simulink model "RLC3rdOrder"  (R2023b)
settings: Solver=VariableStepAuto  StartTime=0.0  StopTime=10.0  RelTol=1e-3
values from neighbouring files (symbols this model uses):
  C = 15    [SimScript.m]
  E = 575    [SimScript.m]
  Kd = 33    [SimScript.m]
  Ki = 10    [SimScript.m]
  Kp = 18    [SimScript.m]
  L = 10    [SimScript.m]
  Q = 10000    [SimScript.m]
  Q0 = 0    [SimScript.m]
  R = 100    [SimScript.m]
settings Model: Creator=Owner  LastModifiedBy=Owner

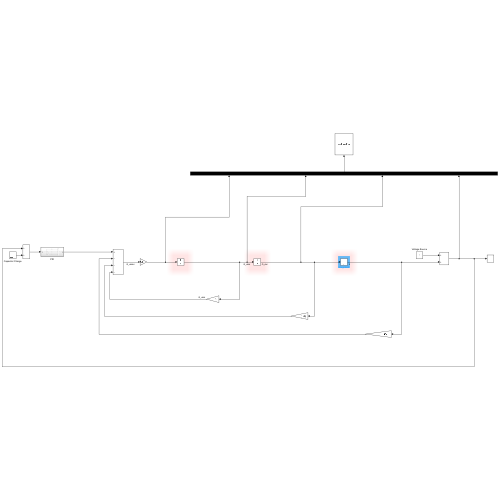
[thumbnail: Simulink's stored preview of the top-level diagram]
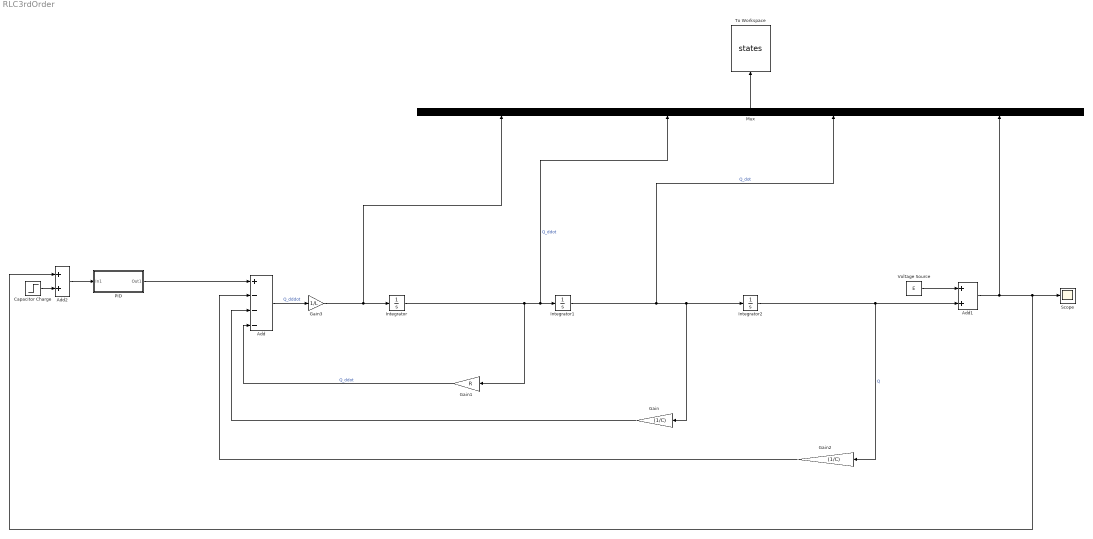
== system RLC3rdOrder ==
  Add : Sum  Inputs=+---
  Add1 : Sum
  Add2 : Sum
  Capacitor Charge : Step  After=Q  SampleTime=0
  Gain : Gain  Gain=(1/C)
  Gain1 : Gain  Gain=R
  Gain2 : Gain  Gain=(1/C)
  Gain3 : Gain  Gain=1/L
  Integrator : Integrator  InitialCondition=Q0
  Integrator1 : Integrator  InitialCondition=Q0
  Integrator2 : Integrator  InitialCondition=Q0
  Mux : Mux
  PID : Subsystem
  Scope : Scope
  To Workspace : ToWorkspace  VariableName=states  SaveFormat=Timeseries  SampleTime=-1
  Voltage Source : Constant  Value=E
  wires:
  Capacitor Charge/1 -> Add2/2
  Add/1 -> Gain3/1  "Q_dddot"
  Integrator/1 -> Mux/2, Integrator1/1, Gain1/1  "Q_ddot"
  Integrator1/1 -> Mux/3, Gain/1, Integrator2/1  "Q_dot"
  Integrator2/1 -> Gain2/1, Add1/2  "Q"
  Voltage Source/1 -> Add1/1
  Add1/1 -> Add2/1, Scope/1, Mux/4
  Gain/1 -> Add/3
  Gain2/1 -> Add/2
  Gain1/1 -> Add/4  "Q_ddot"
  PID/1(Out1) -> Add/1
  Add2/1 -> PID/1(In1)
  Gain3/1 -> Mux/1, Integrator/1
  Mux/1 -> To Workspace/1

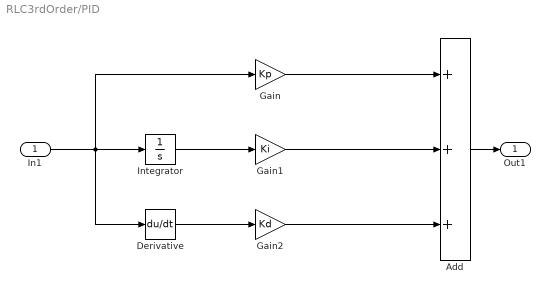
== system RLC3rdOrder/PID ==
  In1 : Inport
  Add : Sum  Inputs=+++
  Derivative : Derivative
  Gain : Gain  Gain=Kp
  Gain1 : Gain  Gain=Ki
  Gain2 : Gain  Gain=Kd
  Integrator : Integrator
  Out1 : Outport
  wires:
  In1/1 -> Derivative/1, Integrator/1, Gain/1
  Integrator/1 -> Gain1/1
  Derivative/1 -> Gain2/1
  Gain/1 -> Add/1
  Gain1/1 -> Add/2
  Gain2/1 -> Add/3
  Add/1 -> Out1/1
